simulink model "sampleModel179"  (R2021b)
settings: Solver=VariableStepAuto  StartTime=0.0  StopTime=10.0  RelTol=1e-3
undefined symbols (not defined in the file or in its folder): DiscIntNeverNeededParam, Newton, Raphson
libraries: simulink x10, slpidlib x1
settings Model: Creator=user  LastModifiedBy=user

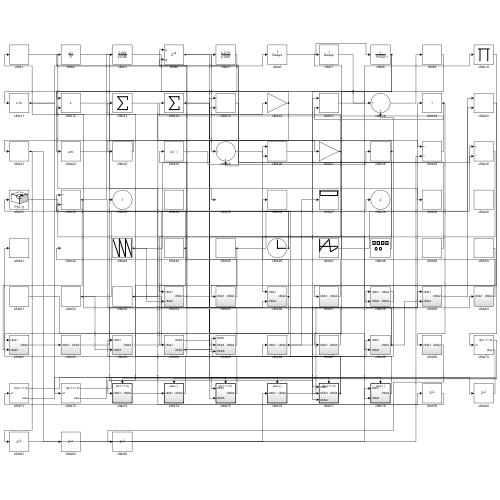
[thumbnail: Simulink's stored preview of the top-level diagram]
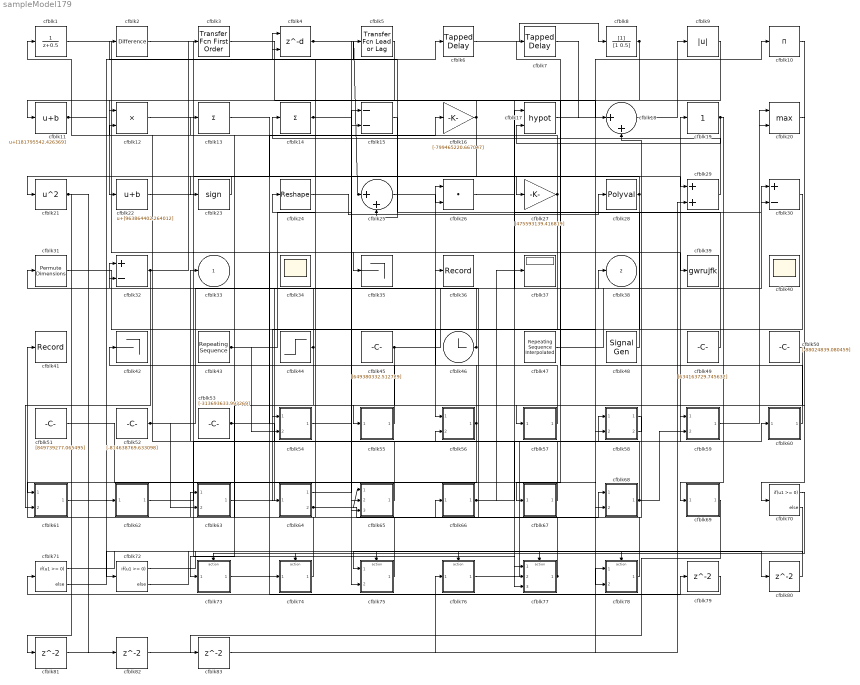
== system sampleModel179 ==
  cfblk1 : DiscreteTransferFcn  SampleTime=1
  cfblk10 : Product  Inputs=*
  cfblk11 : Bias  Bias=[181795542.426369]
  cfblk12 : Product  Inputs=**
  cfblk13 : Sum  Inputs=+
  cfblk14 : Sum  Inputs=+
  cfblk15 : Sum  Inputs=--
  cfblk16 : Gain  Gain=[-799465220.667047]
  cfblk17 : Math  Operator=hypot  SaturateOnIntegerOverflow=on
  cfblk18 : Sum  Inputs=|++
  cfblk19 : simulink/Math Operations/Slider Gain  gain=1  low=0  high=2
  cfblk2 : simulink/Discrete/Difference  ICPrevInput=0.0  OutMin=[]  OutMax=[]  OutDataTypeStr=Inherit: Inherit via back propagation  OutDataType=fixdt(1, 16)  OutScaling=2^-10  DoSatur=off
  cfblk20 : MinMax  Function=max  Inputs=2
  cfblk21 : Math  Operator=square  SaturateOnIntegerOverflow=on
  cfblk22 : Bias  Bias=[963864402.264012]
  cfblk23 : Signum
  cfblk24 : Reshape
  cfblk25 : Sum  Inputs=|++
  cfblk26 : DotProduct  InputSameDT=on  OutDataTypeStr=Inherit: Inherit via internal rule
  cfblk27 : Gain  Gain=[475593139.416819]
  cfblk28 : Polyval  Coefs=[ +2.081618890e-019, -1.441693666e-014, +4.719686976e-010, -8.536869453e-006, +1.621573104e-001, -8.087801117e+001 ]
  cfblk29 : Sum
  cfblk3 : simulink/Discrete/Transfer Fcn First Order  PoleZ=0.95  ICPrevOutput=0.0  DoSatur=off
  cfblk30 : Sum  Inputs=+-
  cfblk31 : PermuteDimensions
  cfblk32 : Sum  Inputs=+-
  cfblk34 : Scope
      settings: Floating=on
  cfblk35 : Terminator
  cfblk36 : Record  FileSettingsInternal="{\"entries\":[{\"content\":{\"excelSettings\":{\"content\":{},\"type\":\"Streamout.ExcelSettings\"}},\"type\":\"Streamout.FileSettingStorage\",\"uuid\":\"2fe2889c-804a-4648-bb93-64e9664d122d\"}],\"packageUris\":[\"http://schema.mathworks.com/mf0/streamout_blocks/R2020a\"],\"version\":\"1.0\"}"  SignalsInternal="{\"entries\":[{\"content\":{\"signals\":[{\"content\":{\"blockPath\":[\"sampleModel179/cfblk36\"],\"channel\":[],\"dimensions\":[1],\"domain\":\"sampleModel179/cfblk36\",\"lineColor\":\"#ff13a6\",\"plots\":[1],\"port\":1,\"sid\":[\"\"],\"signalID\":6697,\"signalName\":\"cfblk77\"},\"type\":\"RecordBlkView.Signal\",\"uuid\":\"7f344007-fab9-4968-983a-89d047d2587d\"}]},\"type\":\"RecordBlkView.InputSignals\",\"uuid\":\"faf1bb9f-562f-42bd-8fab-4d369fa96a04\"}],\"packageUris\":[\"http://schema.mathworks.com/mf0/streamout_blocks/R2020a\"],\"version\":\"1.0\"}"  VisualizationBindings="{\"sparklinesplugin\":{\"info\":[{\"bindingParametersList\":[],\"subplotID\":1}]}}"
  cfblk37 : Display
  cfblk39 : ToWorkspace  VariableName=gwrujfk  SaveFormat=Timeseries  SampleTime=-1
  cfblk4 : Delay  DelayLengthSource=Input port  SampleTime=1
      settings: InputPortMap=u0,p1
  cfblk40 : Scope
      settings: Floating=on
  cfblk41 : Record  FileSettingsInternal="{\"entries\":[{\"content\":{\"excelSettings\":{\"content\":{},\"type\":\"Streamout.ExcelSettings\"}},\"type\":\"Streamout.FileSettingStorage\",\"uuid\":\"5e3a910e-3505-4596-9b85-21d1496942e4\"}],\"packageUris\":[\"http://schema.mathworks.com/mf0/streamout_blocks/R2020a\"],\"version\":\"1.0\"}"  SignalsInternal="{\"entries\":[{\"content\":{\"signals\":[{\"content\":{\"blockPath\":[\"sampleModel179/cfblk41\"],\"channel\":[],\"dimensions\":[1,1],\"domain\":\"sampleModel179/cfblk41\",\"lineColor\":\"#fe330a\",\"plots\":[1],\"port\":1,\"sid\":[\"\"],\"signalID\":6701,\"signalName\":\"cfblk78\"},\"type\":\"RecordBlkView.Signal\",\"uuid\":\"4bde34a3-be9b-4ccf-99bc-c358328e6481\"}]},\"type\":\"RecordBlkView.InputSignals\",\"uuid\":\"60437584-c26f-4991-91f2-ff35db6c0842\"}],\"packageUris\":[\"http://schema.mathworks.com/mf0/streamout_blocks/R2020a\"],\"version\":\"1.0\"}"  VisualizationBindings="{\"sparklinesplugin\":{\"info\":[{\"bindingParametersList\":[],\"subplotID\":1}]}}"
  cfblk42 : Terminator
  cfblk43 : simulink/Sources/Repeating Sequence  rep_seq_t=[0 2]  rep_seq_y=[354312488.790342, -695731924.563452]
  cfblk44 : Step  Time=[32.000000]  Before=[50738360.582872]  After=[399744739.376699]  SampleTime=0
  cfblk45 : Constant  Value=[649380332.512729]  SampleTime=1
  cfblk46 : Clock
  cfblk47 : simulink/Sources/Repeating Sequence Interpolated  OutValues=[-526833701.534994, -147499603.168926, 974237507.540561, -718892622.627222, -124092555.686421]  TimeValues=[0 0.1 0.5 0.6 1].'  LookUpMeth=Use Input Below  tsamp=0.01  OutMin=[]  OutMax=[]  OutDataTypeStr=double  OutputDataTypeScalingMode=double  OutDataType=fixdt(0,8)  OutScaling=2^-10
  cfblk48 : SignalGenerator  WaveForm=sawtooth  Amplitude=[-944307267.684464]  Units=rad/sec
  cfblk49 : Constant  Value=[634163729.745632]  SampleTime=1
  cfblk5 : simulink/Discrete/Transfer Fcn Lead or Lag  PoleZ=0.95  ZeroZ=0.75  ICPrevOutput=0.0  ICPrevInput=0.0  DoSatur=off
      settings: SourceProductBaseCode=SL
  cfblk50 : Constant  Value=[-88024839.080459]  SampleTime=1
  cfblk51 : Constant  Value=[849739277.065495]  SampleTime=1
  cfblk52 : Constant  Value=[-814638769.633098]  SampleTime=1
  cfblk53 : Constant  Value=[-313693633.993269]  SampleTime=1
  cfblk54 : Subsystem
  cfblk55 : Subsystem
  cfblk56 : Subsystem
  cfblk57 : Subsystem
  cfblk58 : Subsystem
  cfblk59 : Subsystem
  cfblk6 : simulink/Discrete/Tapped Delay  vinit=0.0  samptime=-1  NumDelays=1  DelayOrder=Oldest  includeCurrent=off
  cfblk60 : Subsystem
  cfblk61 : Subsystem
  cfblk62 : Subsystem
  cfblk63 : Subsystem
  cfblk64 : Subsystem
  cfblk65 : Subsystem
  cfblk66 : Subsystem
  cfblk67 : Subsystem
  cfblk68 : Subsystem
  cfblk69 : Subsystem
  cfblk7 : simulink/Discrete/Tapped Delay  vinit=0.0  samptime=-1  NumDelays=1  DelayOrder=Oldest  includeCurrent=off
  cfblk70 : If  IfExpression=u1 >= 0  SampleTime=1
  cfblk71 : If  IfExpression=u1 >= 0  SampleTime=1
  cfblk72 : If  IfExpression=u1 >= 0  SampleTime=1
  cfblk73 : Subsystem  TreatAsAtomicUnit=on
  cfblk74 : Subsystem  TreatAsAtomicUnit=on
  cfblk75 : Subsystem  TreatAsAtomicUnit=on
  cfblk76 : Subsystem  TreatAsAtomicUnit=on
  cfblk77 : Subsystem  TreatAsAtomicUnit=on
  cfblk78 : Subsystem  TreatAsAtomicUnit=on
  cfblk{79..83} (5 alike) : Delay  SampleTime=1
  cfblk8 : DiscreteFilter  SampleTime=1
  cfblk9 : Abs
  cfblk33 : Outport
  cfblk38 : Outport  Port=2
  wires:
  cfblk29/1 -> cfblk14/1
  cfblk12/1 -> cfblk27/1
  cfblk52/1 -> cfblk30/1, cfblk63/2(cfblk3)
  cfblk16/1 -> cfblk11/1, cfblk65/3(cfblk5)
  cfblk68/1(cfblk2) -> cfblk58/1(cfblk1), cfblk12/2, cfblk59/2(cfblk4)
  cfblk10/1 -> cfblk57/1(cfblk1)
  cfblk63/1(cfblk2) -> cfblk38/1
  cfblk2/1 -> cfblk75/2(cfblk5)
  cfblk50/1 -> cfblk64/1(cfblk1)
  cfblk4/1 -> cfblk25/1, cfblk77/2(cfblk3)
  cfblk24/1 -> cfblk28/1
  cfblk21/1 -> cfblk81/1, cfblk82/1
  cfblk47/1 -> cfblk20/1
  cfblk59/1(cfblk2) -> cfblk20/2
  cfblk7/1 -> cfblk18/1
  cfblk58/1(cfblk2) -> cfblk66/1(cfblk1)
  cfblk76/1(cfblk2) -> cfblk19/1
  cfblk55/1(cfblk2) -> cfblk42/1
  cfblk8/1 -> cfblk67/1(cfblk1), cfblk77/3(cfblk4)
  cfblk6/1 -> cfblk8/1
  cfblk66/1(cfblk2) -> cfblk59/1(cfblk1), cfblk37/1
  cfblk23/1 -> cfblk21/1
  cfblk43/1 -> cfblk15/1, cfblk54/2(cfblk4)
  cfblk15/1 -> cfblk25/2
  cfblk62/1(cfblk2) -> cfblk60/1(cfblk1)
  cfblk1/1 -> cfblk35/1
  cfblk64/1(cfblk2) -> cfblk15/2
  cfblk74/1(cfblk2) -> cfblk63/1(cfblk1)
  cfblk9/1 -> cfblk22/1
  cfblk56/1(cfblk2) -> cfblk26/1, cfblk61/1(cfblk1)
  cfblk75/1(cfblk2) -> cfblk13/1
  cfblk46/1 -> cfblk31/1, cfblk32/2
  cfblk65/1(cfblk2) -> cfblk33/1
  cfblk20/1 -> cfblk70/1
  cfblk26/1 -> cfblk30/2
  cfblk67/1(cfblk2) -> cfblk4/1
  cfblk78/1(cfblk2) -> cfblk41/1
  cfblk11/1 -> cfblk62/1(cfblk1), cfblk6/1
  cfblk64/2(cfblk5) -> cfblk65/1(cfblk1), cfblk68/1(cfblk1)
  cfblk14/1 -> cfblk39/1, cfblk68/2(cfblk5)
  cfblk61/1(cfblk2) -> cfblk72/1
  cfblk27/1 -> cfblk56/1(cfblk1), cfblk1/1
  cfblk32/1 -> cfblk3/1, cfblk61/2(cfblk5)
  cfblk13/1 -> cfblk29/1
  cfblk45/1 -> cfblk17/1, cfblk55/1(cfblk1)
  cfblk5/1 -> cfblk12/1
  cfblk51/1 -> cfblk77/1(cfblk1)
  cfblk3/1 -> cfblk58/2(cfblk4)
  cfblk30/1 -> cfblk54/1(cfblk1)
  cfblk44/1 -> cfblk73/1(cfblk1), cfblk32/1
  cfblk58/2(cfblk5) -> cfblk18/2
  cfblk31/1 -> cfblk78/2(cfblk4)
  cfblk48/1 -> cfblk5/1
  cfblk18/1 -> cfblk9/1
  cfblk22/1 -> cfblk74/1(cfblk1)
  cfblk53/1 -> cfblk16/1, cfblk56/2(cfblk3)
  cfblk57/1(cfblk2) -> cfblk4/2
  cfblk25/1 -> cfblk26/2
  cfblk28/1 -> cfblk23/1, cfblk65/2(cfblk4)
  cfblk77/1(cfblk2) -> cfblk24/1, cfblk36/1
  cfblk49/1 -> cfblk2/1
  cfblk60/1(cfblk2) -> cfblk7/1
  cfblk17/1 -> cfblk10/1
  cfblk19/1 -> cfblk17/2, cfblk69/1(cfblk1)
  cfblk70/1 -> cfblk73/Action
  cfblk70/2 -> cfblk74/Action
  cfblk71/1 -> cfblk75/Action
  cfblk71/2 -> cfblk76/Action
  cfblk72/1 -> cfblk77/Action
  cfblk72/2 -> cfblk78/Action
  cfblk73/1(cfblk2) -> cfblk79/1
  cfblk79/1 -> cfblk71/1
  cfblk54/1(cfblk2) -> cfblk80/1
  cfblk80/1 -> cfblk75/1(cfblk1)
  cfblk81/1 -> cfblk78/1(cfblk1)
  cfblk82/1 -> cfblk29/2
  cfblk69/1(cfblk2) -> cfblk83/1
  cfblk83/1 -> cfblk76/1(cfblk1)

== system sampleModel179/cfblk54 ==
  cfblk1 : Inport
  cfblk4 : Inport  Port=2
  cfblk3 : Rounding
  cfblk2 : Outport
  wires:
  cfblk4/1 -> cfblk3/1
  cfblk1/1 -> cfblk2/1

== system sampleModel179/cfblk55 ==
  cfblk1 : Inport
  cfblk3 : Constant  Value=[-976285946.988395]  SampleTime=1
  cfblk2 : Outport
  wires:
  cfblk1/1 -> cfblk2/1

== system sampleModel179/cfblk56 ==
  cfblk1 : Inport
  cfblk3 : Inport  Port=2
  cfblk2 : Outport
  wires:
  cfblk3/1 -> cfblk2/1

== system sampleModel179/cfblk57 ==
  cfblk1 : Inport
  cfblk3 : PermuteDimensions
  cfblk2 : Outport
  wires:
  cfblk3/1 -> cfblk2/1
  cfblk1/1 -> cfblk3/1

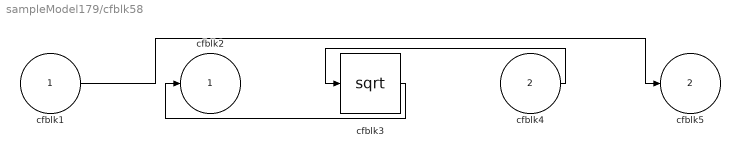
== system sampleModel179/cfblk58 ==
  cfblk1 : Inport
  cfblk4 : Inport  Port=2
  cfblk3 : Sqrt  SaturateOnIntegerOverflow=on
  cfblk2 : Outport
  cfblk5 : Outport  Port=2
  wires:
  cfblk4/1 -> cfblk3/1
  cfblk3/1 -> cfblk2/1
  cfblk1/1 -> cfblk5/1

== system sampleModel179/cfblk59 ==
  cfblk1 : Inport
  cfblk4 : Inport  Port=2
  cfblk3 : Polyval  Coefs=[ +2.081618890e-019, -1.441693666e-014, +4.719686976e-010, -8.536869453e-006, +1.621573104e-001, -8.087801117e+001 ]
  cfblk2 : Outport
  wires:
  cfblk1/1 -> cfblk2/1
  cfblk4/1 -> cfblk3/1

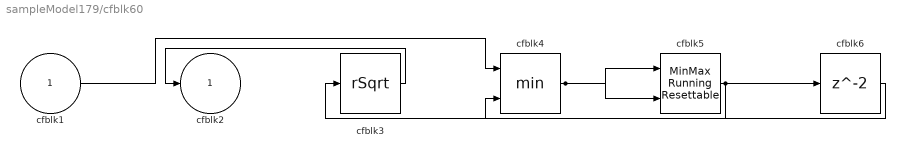
== system sampleModel179/cfblk60 ==
  cfblk1 : Inport
  cfblk3 : Sqrt  Operator=rSqrt  AlgorithmType=Newton-Raphson  SaturateOnIntegerOverflow=on
  cfblk4 : MinMax  Inputs=2
  cfblk5 : simulink/Math Operations/MinMax Running Resettable  Function=min  vinit=0.0
  cfblk6 : Delay  SampleTime=1
  cfblk2 : Outport
  wires:
  cfblk3/1 -> cfblk2/1
  cfblk4/1 -> cfblk5/1, cfblk5/2
  cfblk1/1 -> cfblk4/1
  cfblk5/1 -> cfblk3/1, cfblk6/1
  cfblk6/1 -> cfblk4/2

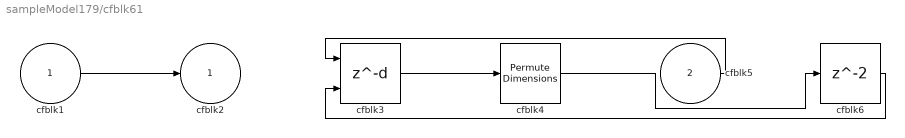
== system sampleModel179/cfblk61 ==
  cfblk1 : Inport
  cfblk5 : Inport  Port=2
  cfblk3 : Delay  DelayLengthSource=Input port  SampleTime=1
      settings: InputPortMap=u0,p1
  cfblk4 : PermuteDimensions
  cfblk6 : Delay  SampleTime=1
  cfblk2 : Outport
  wires:
  cfblk3/1 -> cfblk4/1
  cfblk5/1 -> cfblk3/1
  cfblk1/1 -> cfblk2/1
  cfblk4/1 -> cfblk6/1
  cfblk6/1 -> cfblk3/2

== system sampleModel179/cfblk62 ==
  cfblk1 : Inport
  cfblk3 : simulink/Discrete/Difference  ICPrevInput=0.0  OutMin=[]  OutMax=[]  OutDataTypeStr=Inherit: Inherit via back propagation  OutDataType=fixdt(1, 16)  OutScaling=2^-10  DoSatur=off
  cfblk2 : Outport
  wires:
  cfblk1/1 -> cfblk3/1
  cfblk3/1 -> cfblk2/1

== system sampleModel179/cfblk63 ==
  cfblk1 : Inport
  cfblk3 : Inport  Port=2
  cfblk2 : Outport
  wires:
  cfblk3/1 -> cfblk2/1

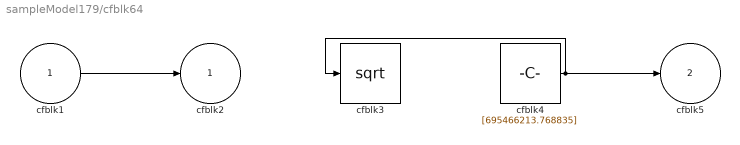
== system sampleModel179/cfblk64 ==
  cfblk1 : Inport
  cfblk3 : Sqrt  SaturateOnIntegerOverflow=on
  cfblk4 : Constant  Value=[695466213.768835]  SampleTime=1
  cfblk2 : Outport
  cfblk5 : Outport  Port=2
  wires:
  cfblk4/1 -> cfblk5/1, cfblk3/1
  cfblk1/1 -> cfblk2/1

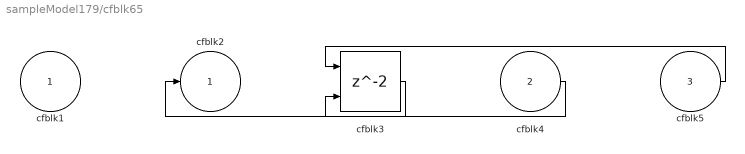
== system sampleModel179/cfblk65 ==
  cfblk1 : Inport
  cfblk4 : Inport  Port=2
  cfblk5 : Inport  Port=3
  cfblk3 : Delay  ShowEnablePort=on  SampleTime=1
      settings: InputPortMap=u0,e6
  cfblk2 : Outport
  wires:
  cfblk5/1 -> cfblk3/1
  cfblk3/1 -> cfblk2/1
  cfblk4/1 -> cfblk3/2

== system sampleModel179/cfblk66 ==
  cfblk1 : Inport
  cfblk3 : Sum  Inputs=+-
  cfblk2 : Outport
  wires:
  cfblk1/1 -> cfblk2/1, cfblk3/1, cfblk3/2

== system sampleModel179/cfblk67 ==
  cfblk1 : Inport
  cfblk3 : Rounding
  cfblk2 : Outport
  wires:
  cfblk1/1 -> cfblk3/1
  cfblk3/1 -> cfblk2/1

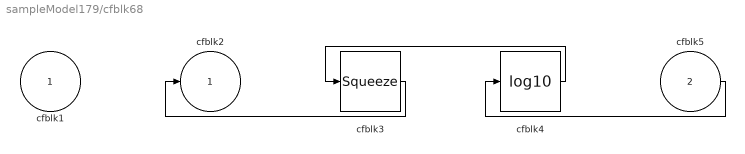
== system sampleModel179/cfblk68 ==
  cfblk1 : Inport
  cfblk5 : Inport  Port=2
  cfblk3 : Squeeze
  cfblk4 : Math  Operator=log10  SaturateOnIntegerOverflow=on
  cfblk2 : Outport
  wires:
  cfblk4/1 -> cfblk3/1
  cfblk3/1 -> cfblk2/1
  cfblk5/1 -> cfblk4/1

== system sampleModel179/cfblk69 ==
  cfblk1 : Inport
  cfblk3 : DiscreteIntegrator  ICPrevOutput=DiscIntNeverNeededParam  ICPrevScaledInput=DiscIntNeverNeededParam
  cfblk2 : Outport
  wires:
  cfblk1/1 -> cfblk3/1
  cfblk3/1 -> cfblk2/1

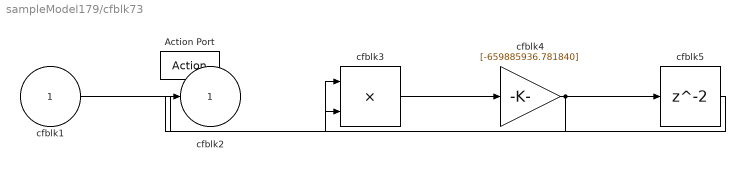
== system sampleModel179/cfblk73 ==
  cfblk1 : Inport
  Action Port : ActionPort  ActionPortLabel=if(u1 >= 0)
  cfblk3 : Product
  cfblk4 : Gain  Gain=[-659885936.781840]
  cfblk5 : Delay
  cfblk2 : Outport
  wires:
  cfblk1/1 -> cfblk3/1
  cfblk3/1 -> cfblk4/1
  cfblk4/1 -> cfblk2/1, cfblk5/1
  cfblk5/1 -> cfblk3/2

== system sampleModel179/cfblk74 ==
  cfblk1 : Inport
  Action Port : ActionPort  ActionPortLabel=else
  cfblk3 : Constant  Value=[-541020629.266397]  SampleTime=1
  cfblk2 : Outport
  wires:
  cfblk1/1 -> cfblk2/1

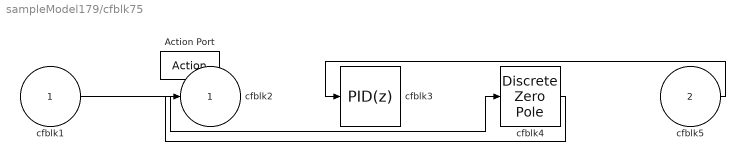
== system sampleModel179/cfblk75 ==
  cfblk1 : Inport
  cfblk5 : Inport  Port=2
  Action Port : ActionPort  ActionPortLabel=if(u1 >= 0)
  cfblk3 : slpidlib/PID Controller  Controller=PID  Form=Parallel  TimeDomain=Discrete-time  UseExternalTs=off  SampleTime=-1  IntegratorMethod=Forward Euler  FilterMethod=Forward Euler  ControllerParametersSource=internal  P=1  I=1  D=0  UseFilter=on  N=100  TunerSelectOption=Transfer Function Based (PID Tuner App)  InitialConditionSource=internal  InitialConditionForIntegrator=0  InitialConditionForFilter=0  DifferentiatorICPrevScaledInput=0  ExternalReset=none  TrackingMode=off  Kt=1  LimitOutput=off  SatLimitsSource=internal  UpperSaturationLimit=inf  LowerSaturationLimit=-inf  LinearizeAsGain=off  AntiWindupMode=none  Kb=1  POutMin=[]  POutMax=[]  IOutMin=[]  IOutMax=[]  DOutMin=[]  DOutMax=[]  NOutMin=[]  NOutMax=[]  SumOutMin=[]  SumOutMax=[]  SaturationOutMin=[]  SaturationOutMax=[]  PParamMin=[]  PParamMax=[]  IParamMin=[]  IParamMax=[]  DParamMin=[]  DParamMax=[]  NParamMin=[]  NParamMax=[]  KbParamMin=[]  KbParamMax=[]  KtParamMin=[]  KtParamMax=[]  KbOutMin=[]  KbOutMax=[]  KtOutMin=[]  KtOutMax=[]  IntegratorOutMin=[]  IntegratorOutMax=[]  FilterOutMin=[]  FilterOutMax=[]  SumI1OutMin=[]  SumI1OutMax=[]  SumI2OutMin=[]  SumI2OutMax=[]  SumI3OutMin=[]  SumI3OutMax=[]  SumI4OutMin=[]  SumI4OutMax=[]  SumDOutMin=[]  SumDOutMax=[]  DifferentiatorOutMin=[]  DifferentiatorOutMax=[]  FilterDiffOutCoefMin=[]  FilterDiffOutCoefMax=[]  ReciprocalOutMin=[]  ReciprocalOutMax=[]  SumDenOutMin=[]  SumDenOutMax=[]  SumNumOutMin=[]  SumNumOutMax=[]  DivideOutMin=[]  DivideOutMax=[]  UdiffTsProdOutMin=[]  UdiffTsProdOutMax=[]  NTsProdOutMin=[]  NTsProdOutMax=[]  UintegralTsProdOutMin=[]  UintegralTsProdOutMax=[]  UngainTsProdOutMin=[]  UngainTsProdOutMax=[]  IntegratorContinuousStateAttributes=''  IntegratorStateMustResolveToSignalObject=off  IntegratorRTWStateStorageClass=Auto  FilterContinuousStateAttributes=''  FilterStateMustResolveToSignalObject=off  FilterRTWStateStorageClass=Auto  ParallelPVariant=InternalParameters  IdealPVariant=Disabled  IVariant=InternalParameters  DVariant=InternalParameters  IntegratorVariant=Discrete  SatVariant=Disabled  AWVariant=Passthrough  PCopyVariant=Disabled  TRVariant=Disabled  FdbkBlocksVariant=Forward  IdealPFdbkVariant=Disabled  SatFdbkVariant=Disabled  DerivativeFilterVariant=ForwardEulerFilter  NVariant=InternalParameters  NCopyVariant=Disabled  FilterICVariant=InternalICsFilter  IntegratorICVariant=InternalICs  ExternalResetVariant=Disabled  TRSumVariant=Passthrough  SumFdbkVariant=Disabled  SumVariant=Sum_PID  TsampFilterVariant=InternalTs  TsampNgainVariant=Passthrough  TsampIntegralVariant=Passthrough  ExternalSaturationOutDataTypeStr=Inherit: Same as second input
  cfblk4 : DiscreteZeroPole  Poles=[0 0.5]  Gain=1  SampleTime=-1
  cfblk2 : Outport
  wires:
  cfblk1/1 -> cfblk4/1
  cfblk4/1 -> cfblk2/1
  cfblk5/1 -> cfblk3/1

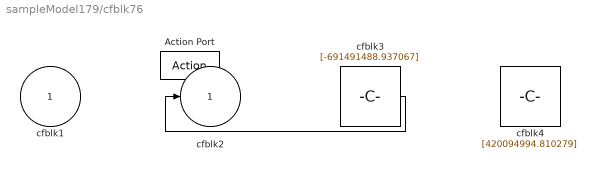
== system sampleModel179/cfblk76 ==
  cfblk1 : Inport
  Action Port : ActionPort  ActionPortLabel=else
  cfblk3 : Constant  Value=[-691491488.937067]  SampleTime=1
  cfblk4 : Constant  Value=[420094994.810279]  SampleTime=1
  cfblk2 : Outport
  wires:
  cfblk3/1 -> cfblk2/1

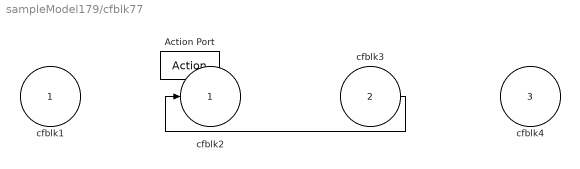
== system sampleModel179/cfblk77 ==
  cfblk1 : Inport
  cfblk3 : Inport  Port=2
  cfblk4 : Inport  Port=3
  Action Port : ActionPort  ActionPortLabel=if(u1 >= 0)
  cfblk2 : Outport
  wires:
  cfblk3/1 -> cfblk2/1

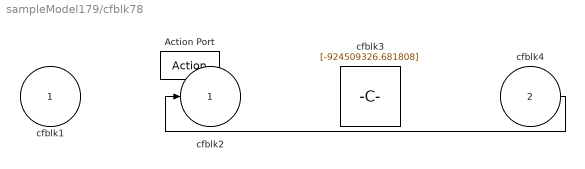
== system sampleModel179/cfblk78 ==
  cfblk1 : Inport
  cfblk4 : Inport  Port=2
  Action Port : ActionPort  ActionPortLabel=else
  cfblk3 : Constant  Value=[-924509326.681808]  SampleTime=1
  cfblk2 : Outport
  wires:
  cfblk4/1 -> cfblk2/1
